simulink model "projeto_garra_1"  (R2024b)
settings: Solver=FixedStepAuto  StartTime=0.0  StopTime=10.0  RelTol=1e-3
model workspace (MAT data in the model file):
  SL_ROS_VariableLengthArrays_MaxSizes.CommonInfo.ArrayTruncateAction = 'EmitWarning'
  SL_ROS_VariableLengthArrays_MaxSizes.MsgTypeMap = containers.Map
  SL_ROS_VariableLengthArrays_MaxSizes.MsgTypeMap.serialization.keys = {'trajectory_msgs/JointTrajectory'}
  SL_ROS_VariableLengthArrays_MaxSizes.MsgTypeMap.serialization.values{1}(1).PropertyName = 'JointNames'
  SL_ROS_VariableLengthArrays_MaxSizes.MsgTypeMap.serialization.values{1}(1).DataType = 'std_msgs/String'
  SL_ROS_VariableLengthArrays_MaxSizes.MsgTypeMap.serialization.values{1}(1).MaxLength = 16
  SL_ROS_VariableLengthArrays_MaxSizes.MsgTypeMap.serialization.values{1}(2).PropertyName = 'Points'
  SL_ROS_VariableLengthArrays_MaxSizes.MsgTypeMap.serialization.values{1}(2).DataType = 'trajectory_msgs/JointTrajectoryPoint'
  SL_ROS_VariableLengthArrays_MaxSizes.MsgTypeMap.serialization.values{1}(2).MaxLength = 7
  SL_ROS_VariableLengthArrays_MaxSizes.MsgTypeMap.serialization.uniformity = 0
  SL_ROS_VariableLengthArrays_MaxSizes.MsgTypeMap.serialization.keyType = 'char'
  SL_ROS_VariableLengthArrays_MaxSizes.MsgTypeMap.serialization.valueType = 'any'
libraries: robotlib x4
settings Model: ExtModeBatchMode=on  Creator=pecci  LastModifiedBy=pecci
settings OptimizationCC: DefaultParameterBehavior=Inlined  EnhancedBackFolding=on  PassReuseOutputArgsAs=Individual arguments  ZeroExternalMemoryAtStartup=off  ZeroInternalMemoryAtStartup=off  MaxStackSize=64  OptimizeBlockOrder=speed  DifferentSizesBufferReuse=on  OptimizationCustomize=off  EfficientTunableParamExpr=on
settings DebuggingCC: ParameterTunabilityLossMsg=error
settings HardwareCC: ProdBitPerPointer=32  ProdBitPerSizeT=32  ProdBitPerPtrDiffT=32  ProdLargestAtomicFloat=None  ProdIntDivRoundTo=Undefined  ProdEndianess=Unspecified  ProdWordSize=32  ProdHWDeviceType=Generic->Unspecified (assume 32-bit Generic)
settings SFSimCC: MATLABDynamicMemAlloc=off
settings RTWCC: Description=Embedded Coder  SystemTargetFile=ert.tlc  HardwareBoard=Robot Operating System (ROS)  TLCOptions="-aInlineSetEventsForThisBaseRateFcn=TLC_FALSE -aSuppressMultiTaskScheduler=TLC_FALSE  -aRateBasedStepFcn=0"  TemplateMakefile=ert_default_tmf  Toolchain=Catkin  TargetLang=C++
settings CodeAppCC: ForceParamTrailComments=on  IgnoreCustomStorageClasses=off  OperatorAnnotations=on  SimulinkDataObjDesc=on  SFDataObjDesc=on  InsertBlockDesc=on

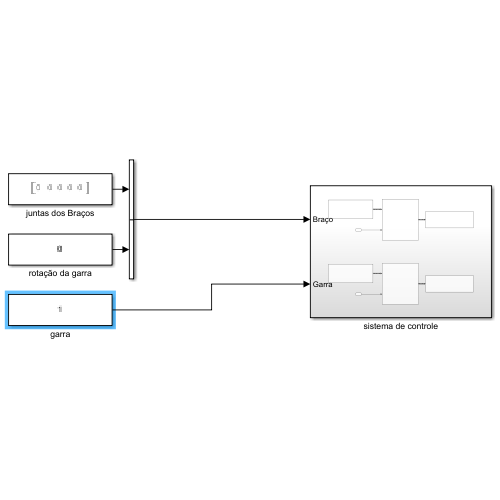
[thumbnail: Simulink's stored preview of the top-level diagram]
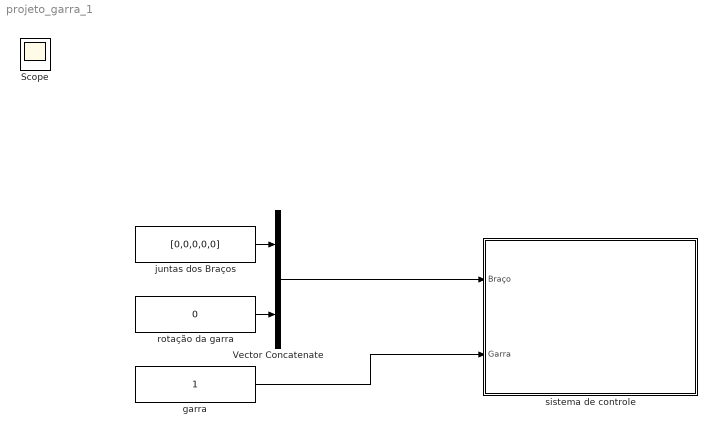
== system projeto_garra_1 ==
  Vector Concatenate : Concatenate
  garra : Constant
  juntas dos Braços : Constant  Value=[0,0,0,0,0]
  rotação da garra : Constant  Value=0
  sistema de controle : Subsystem
  Scope : Scope
  wires:
  garra/1 -> sistema de controle/2(Garra)
  juntas dos Braços/1 -> Vector Concatenate/1
  rotação da garra/1 -> Vector Concatenate/2
  Vector Concatenate/1 -> sistema de controle/1(Braço)

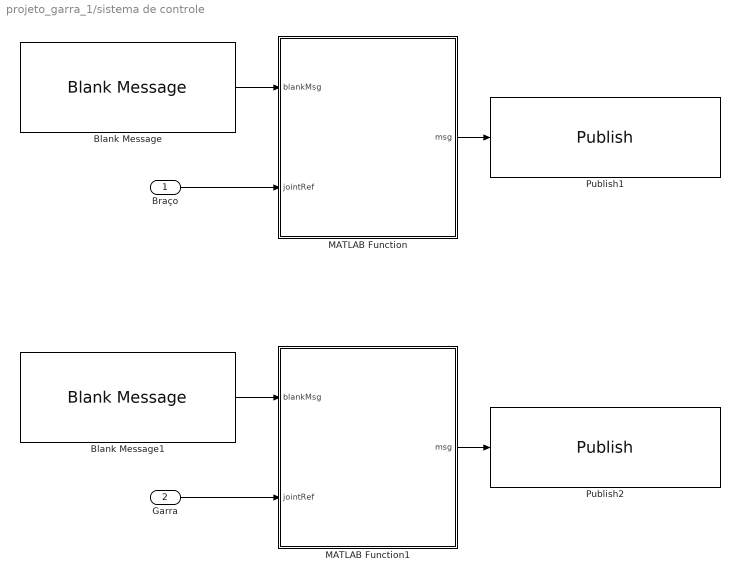
== system projeto_garra_1/sistema de controle ==
  Braço : Inport
  Garra : Inport  Port=2
  Blank Message : robotlib/Blank Message  messageClass=Message  entityType=trajectory_msgs/JointTrajectory  messageType=trajectory_msgs/JointTrajectory  SampleTime=inf  legacyBusStruct=off
  Blank Message1 : robotlib/Blank Message  messageClass=Message  entityType=trajectory_msgs/JointTrajectory  messageType=trajectory_msgs/JointTrajectory  SampleTime=inf  legacyBusStruct=off
  MATLAB Function : MATLAB Function  TreatAsAtomicUnit=on
  MATLAB Function1 : MATLAB Function  TreatAsAtomicUnit=on
  Publish1 : robotlib/Publish  topicSource=Select from ROS network  topic=/pos_joint_traj_controller/command  messageType=trajectory_msgs/JointTrajectory  legacyBusStruct=off  messageQueueLength=1
  Publish2 : robotlib/Publish  topicSource=Select from ROS network  topic=/gripper_controller/command  messageType=trajectory_msgs/JointTrajectory  legacyBusStruct=off  messageQueueLength=1
  wires:
  Blank Message1/1 -> MATLAB Function1/1(blankMsg)
  Blank Message/1 -> MATLAB Function/1(blankMsg)
  MATLAB Function/1(msg) -> Publish1/1
  Garra/1 -> MATLAB Function1/2(jointRef)
  Braço/1 -> MATLAB Function/2(jointRef)
  MATLAB Function1/1(msg) -> Publish2/1

== matlab function projeto_garra_1/sistema de controle/MATLAB Function1 ==
  data: blankMsg input; msg output Bus: SL_Bus_simulinkros_braco_1_trajectory_msgs_JointTrajectory; jointRef input
function msg = packageTrajectory(blankMsg, jointRef)

    msg = blankMsg;

    
    numJoints = uint32(1);
    msg.JointNames_SL_Info.CurrentLength = numJoints;

  
    name = 'robotiq_85_left_knuckle_joint';
    msg.JointNames(1).Data(1:length(name)) = uint8(name);
    msg.JointNames(1).Data_SL_Info.CurrentLength = uint32(length(name));

    msg.Points_SL_Info.CurrentLength = uint32(1);

    msg.Points(1).TimeFromStart.Sec = 1;
    msg.Points(1).TimeFromStart.Nsec = 0;

    msg.Points(1).Positions_SL_Info.CurrentLength = numJoints;
    msg.Points(1).Positions(1:numJoints) = jointRef;

    msg.Points(1).Velocities_SL_Info.CurrentLength = numJoints;
    msg.Points(1).Velocities(1:numJoints) = zeros(numJoints,1);

    msg.Points(1).Accelerations_SL_Info.CurrentLength = numJoints;
    msg.Points(1).Accelerations(1:numJoints) = zeros(numJoints,1);

    msg.Points(1).Effort_SL_Info.CurrentLength = numJoints;
    msg.Points(1).Effort(1:numJoints) = zeros(numJoints,1);

    % Header com valores padrão
msg.Header.Stamp.Sec = 0;
msg.Header.Stamp.Nsec = 0;
msg.Header.Seq = uint32(1);
msg.Header.FrameId = uint8(zeros(128,1));  % força 1x128 com transposição
msg.Header.FrameId_SL_Info.CurrentLength = uint32(0);


end

== matlab function projeto_garra_1/sistema de controle/MATLAB Function ==
  data: blankMsg input; msg output Bus: SL_Bus_simulinkros_braco_1_trajectory_msgs_JointTrajectory; jointRef input
function msg = packageTrajectory(blankMsg, jointRef)

    msg = blankMsg;

msg.JointNames_SL_Info.CurrentLength = uint32(6);

msg.JointNames(1).Data_SL_Info.CurrentLength = uint32(18);
msg.JointNames(1).Data(1:18) = uint8('shoulder_pan_joint')';
msg.JointNames(2).Data_SL_Info.CurrentLength = uint32(19);
msg.JointNames(2).Data(1:19) = uint8('shoulder_lift_joint')';
msg.JointNames(3).Data_SL_Info.CurrentLength = uint32(11);
msg.JointNames(3).Data(1:11) = uint8('elbow_joint')';
msg.JointNames(4).Data_SL_Info.CurrentLength = uint32(13);
msg.JointNames(4).Data(1:13) = uint8('wrist_1_joint')';
msg.JointNames(5).Data_SL_Info.CurrentLength = uint32(13);
msg.JointNames(5).Data(1:13) = uint8('wrist_2_joint')';
msg.JointNames(6).Data_SL_Info.CurrentLength = uint32(13);
msg.JointNames(6).Data(1:13) = uint8('wrist_3_joint')';

numJoints = uint32(6);

    msg.Points_SL_Info.CurrentLength = uint32(1);

    msg.Points(1).TimeFromStart.Sec = 1;
    msg.Points(1).TimeFromStart.Nsec = 0;

    msg.Points(1).Positions_SL_Info.CurrentLength = numJoints;
    msg.Points(1).Positions(1:numJoints) = jointRef;

    msg.Points(1).Velocities_SL_Info.CurrentLength = numJoints;
    msg.Points(1).Velocities(1:numJoints) = zeros(numJoints,1);

    msg.Points(1).Accelerations_SL_Info.CurrentLength = numJoints;
    msg.Points(1).Accelerations(1:numJoints) = zeros(numJoints,1);

    msg.Points(1).Effort_SL_Info.CurrentLength = numJoints;
    msg.Points(1).Effort(1:numJoints) = zeros(numJoints,1);

    % Header com valores padrão
msg.Header.Stamp.Sec = 0;
msg.Header.Stamp.Nsec = 0;
msg.Header.Seq = uint32(1);
msg.Header.FrameId = uint8(zeros(128,1));  % força 1x128 com transposição
msg.Header.FrameId_SL_Info.CurrentLength = uint32(0);

end
